simulink model "Testodesto"  (R2025b)
settings: Solver=ode23s  StartTime=0.0  StopTime=50  RelTol=1e-3
values from neighbouring files (symbols this model uses):
  A_sym_calc = sym(A_num)    [calculate_system.m]
  B_sym_calc = sym(B_num)    [calculate_system.m]
  C_sym_calc = sym(C_num)    [calculate_system.m]
settings Model: Creator=fabim  LastModifiedBy=fabim

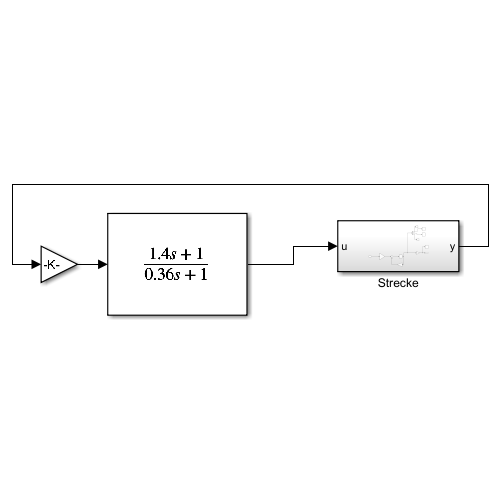
[thumbnail: Simulink's stored preview of the top-level diagram]
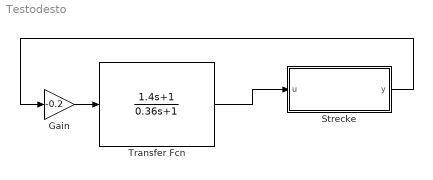
== system Testodesto ==
  Gain : Gain  Gain=-0.2
  Strecke : Subsystem
  Transfer Fcn : TransferFcn  Numerator=[1.4 1]  Denominator=[0.36 1]
  wires:
  Transfer Fcn/1 -> Strecke/1(u)
  Gain/1 -> Transfer Fcn/1
  Strecke/1(y) -> Gain/1

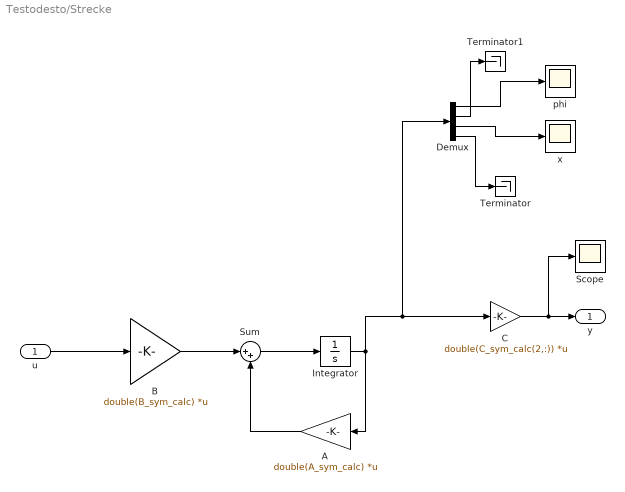
== system Testodesto/Strecke ==
  u : Inport
  A : Gain  Gain=double(A_sym_calc)  Multiplication=Matrix(K*u)
  B : Gain  Gain=double(B_sym_calc)  Multiplication=Matrix(K*u)
  C : Gain  Gain=double(C_sym_calc(2,:))  Multiplication=Matrix(K*u)
  Demux : Demux
  Integrator : Integrator  InitialCondition=[0.1;0;0;0]
  Scope : Scope
      settings: ActiveDisplayYMinimum=-0.096422387436448709  ActiveDisplayYMaximum=0.0692669900128686
  Sum : Sum  Inputs=|++
  Terminator : Terminator
  Terminator1 : Terminator
  phi : Scope
      settings: ActiveDisplayYMinimum=-0.060170355003542994  ActiveDisplayYMaximum=0.072892092984425186
  x : Scope
      settings: ActiveDisplayYMinimum=-0.12609102571146941  ActiveDisplayYMaximum=0.1540604441377027  DataLoggingVariableName=ScopeData2
  y : Outport
  wires:
  Sum/1 -> Integrator/1
  A/1 -> Sum/2
  B/1 -> Sum/1
  u/1 -> B/1
  Integrator/1 -> A/1, Demux/1, C/1
  C/1 -> Scope/1, y/1
  Demux/1 -> phi/1
  Demux/3 -> x/1
  Demux/4 -> Terminator/1
  Demux/2 -> Terminator1/1
